simulink model "model"  (R2018a)
settings: Solver=ode14x  StartTime=0.0  StopTime=10  FixedStep=0.01  RelTol=1e-3
values from neighbouring files (symbols this model uses):
  ioKd = -1.48994791343    [param.mat]
  ioKi = -0.181850602386    [param.mat]
  ioKp = -1.57948118522    [param.mat]
  k = -0.8592    [param.mat]    (also in zz.m = -N:N)
  Ki = 0.882906706311    [param.mat]
  Kp = -1.54891181175    [param.mat]
  Lambda = -0.9885    [param.mat]
  tau = 1.071    [param.mat]
settings Model: Creator=Bo Shang  LastModifiedBy=standard
settings DataIOCC: LimitDataPoints=on  SaveFormat=Array  SaveState=on
settings OptimizationCC: BlockReduction=off  BooleanDataType=off  LifeSpan=inf
settings DebuggingCC: SaveWithParameterizedLinksMsg=none  UnderspecifiedInitializationDetection=Classic  MergeDetectMultiDrivingBlocksExec=none  SignalResolutionControl=TryResolveAllWithWarning  SFUnexpectedBacktrackingDiag=warning  SFNoUnconditionalDefaultTransitionDiag=warning  SFExecutionAtInitializationDiag=none
settings HardwareCC: ProdBitPerPointer=32  ProdBitPerSizeT=32  ProdBitPerPtrDiffT=32  ProdLargestAtomicFloat=None  ProdIntDivRoundTo=Undefined  ProdEndianess=Unspecified  ProdWordSize=32  ProdHWDeviceType=32-bit Generic  TargetUnknown=on
settings ModelReferenceCC: PropagateSignalLabelsOutOfModel=off
settings CodeAppCC: StateflowObjectComments=on
settings GRTTargetCC: TargetLangStandard=C89/C90 (ANSI)  GeneratePreprocessorConditionals=Disable all
settings ConfigComp: CovMetricSettings=dw  CovHtmlReporting=on  CovSaveCumulativeToWorkspaceVar=on  CovSaveSingleToWorkspaceVar=on  CovExternalEMLEnable=off  CovSFcnEnable=off

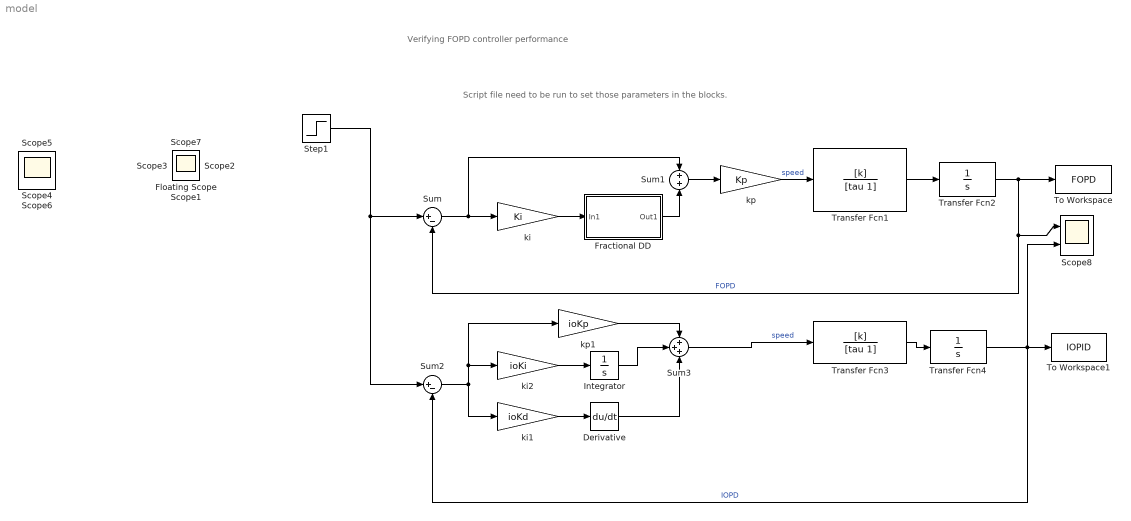
== system model ==
  note: Verifying FOPD controller performance
  note: Script file need to be run to set those parameters in the blocks.
  Derivative : Derivative  CoefficientInTFapproximation=0
  Fractional DD : Subsystem  mask{gam=-Lambda, ww=[0.001,1000], n=4}
      mask prompts: gam "Derivative order gamma"; ww "Frequency range [wb,wh]"; n "Apprixmation order"
      mask init:
      | wb=ww(1); wh=ww(2); G=zz(gam,n,wb,wh);
      | num=G.num{1}; den=G.den{1}; T=1/wh; str='Fractional\n';
      | if isnumeric(gam)
      | 	if gam>0, str=[str, 'Der  s^' num2str(gam) ];
      | 	else, str=[str, 'Int  s^{' num2str(gam) '}']; end
      | else, str=[str, 'Der  s^gam']; end
      mask Display: disp(str)
  Integrator : Integrator
  Scope8 : Scope  NumInputPorts=2
  Step1 : Step  Time=0  SampleTime=0
  Sum : Sum  Inputs=|+-
  Sum1 : Sum  Inputs=+|+
  Sum2 : Sum  Inputs=|+-
  Sum3 : Sum  Inputs=+++
  To Workspace : ToWorkspace  VariableName=FOPD  SaveFormat=Timeseries  SampleTime=-1
  To Workspace1 : ToWorkspace  VariableName=IOPID  SaveFormat=Timeseries  SampleTime=-1
  Transfer Fcn1 : TransferFcn  Numerator=[k]  Denominator=[tau 1]
  Transfer Fcn2 : TransferFcn  Denominator=[1 0]
  Transfer Fcn3 : TransferFcn  Numerator=[k]  Denominator=[tau 1]
  Transfer Fcn4 : TransferFcn  Denominator=[1 0]
  ki : Gain  Gain=Ki
  ki1 : Gain  Gain=ioKd
  ki2 : Gain  Gain=ioKi
  kp : Gain  Gain=Kp
  kp1 : Gain  Gain=ioKp
  Floating Scope : Scope
  Scope{,1..7} (8 alike) : Scope
  wires:
  Fractional DD/1(Out1) -> Sum1/2
  ki/1 -> Fractional DD/1(In1)
  kp/1 -> Transfer Fcn1/1  "speed"
  Sum1/1 -> kp/1
  Sum/1 -> Sum1/1, ki/1
  Transfer Fcn1/1 -> Transfer Fcn2/1
  Transfer Fcn2/1 -> To Workspace/1, Scope8/1, Sum/2  "FOPD"
  Transfer Fcn3/1 -> Transfer Fcn4/1
  Transfer Fcn4/1 -> To Workspace1/1, Scope8/2, Sum2/2  "IOPD"
  Step1/1 -> Sum2/1, Sum/1
  Derivative/1 -> Sum3/3
  ki1/1 -> Derivative/1
  Sum3/1 -> Transfer Fcn3/1  "speed"
  kp1/1 -> Sum3/1
  ki2/1 -> Integrator/1
  Sum2/1 -> kp1/1, ki2/1, ki1/1
  Integrator/1 -> Sum3/2

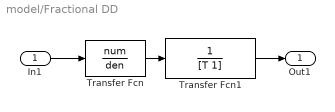
== system model/Fractional DD ==
  In1 : Inport
  Transfer Fcn : TransferFcn  Numerator=num  Denominator=den
  Transfer Fcn1 : TransferFcn  Numerator=1  Denominator=[T 1]
  Out1 : Outport
  wires:
  Transfer Fcn1/1 -> Out1/1
  Transfer Fcn/1 -> Transfer Fcn1/1
  In1/1 -> Transfer Fcn/1
